simulink model "io306"  (Simulink 6.0)
settings: Solver=FixedStepDiscrete  StartTime=0.0  StopTime=4  FixedStep=0.001  RelTol=1e-3
libraries: xpcrealtimedeviceslib x6
settings Model: Creator=pkirwin  LastModifiedBy=ekbas  ExtModeArmWhenConnect=off  BufferReuse=off  ProdHWDeviceType=Specified
settings DataIOCC: SaveFormat=Structure  SignalLoggingName=sigsOut
settings OptimizationCC: BlockReduction=off  BooleanDataType=off  InlineInvariantSignals=off  OptimizeBlockIOStorage=off  BufferReuse=off  EnforceIntegerDowncast=off  FoldNonRolledExpr=off  LocalBlockOutputs=off
settings DebuggingCC: CheckExecutionContextPreStartOutputMsg=on  CheckExecutionContextRuntimeOutputMsg=on  SolverPrmCheckMsg=none
settings HardwareCC: ProdBitPerShort=32  ProdBitPerInt=16  ProdHWDeviceType=Specified  TargetHWDeviceType=32-bit Generic  ProdEqTarget=off
settings RTWCC: SystemTargetFile=xpctarget.tlc  TemplateMakefile=xpc_default_tmf  ProcessScript=xpctarget_make_rtw_hook
settings xpcTargetCC: TargetFcnLib=ansi_tfl_tmw.mat  GenFloatMathFcnCalls=ANSI_C  ModelReferenceCompliant=off
settings SFSimCC: SFSimApplyToAllLibs=on  SFSimBuildMode=Incremental

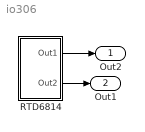
== system io306 ==
  RTD6814 : Subsystem  PropExecContextAcrossSSBoundary=on
  Out2 : Outport
  Out1 : Outport  Port=2
  wires:
  RTD6814/1(Out1) -> Out2/1
  RTD6814/2(Out2) -> Out1/1

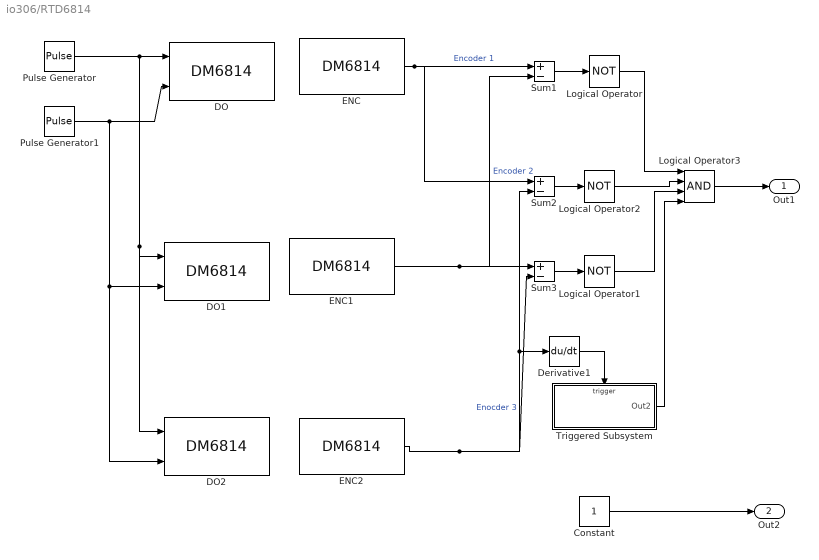
== system io306/RTD6814 ==
  Constant : Constant
  DO : xpcrealtimedeviceslib/Digital Output/DM6814   channel=[1 2]  port=A  reset=[1]  initValue=[0]  sampleTime=.001  baseHex=0x280
  DO1 : xpcrealtimedeviceslib/Digital Output/DM6814   channel=[1 2]  port=B  reset=[1]  initValue=[0]  sampleTime=.001  baseHex=0x280
  DO2 : xpcrealtimedeviceslib/Digital Output/DM6814   channel=[1 2]  port=C  reset=[1]  initValue=[0]  sampleTime=.001  baseHex=0x280
  Derivative1 : Derivative
  ENC : xpcrealtimedeviceslib/Incremental Encoder/DM6814   channel=1  initValue=0  reset=off  sampleTime=0.001  baseHex=0x280
  ENC1 : xpcrealtimedeviceslib/Incremental Encoder/DM6814   channel=2  initValue=0  reset=off  sampleTime=0.001  baseHex=0x280
  ENC2 : xpcrealtimedeviceslib/Incremental Encoder/DM6814   channel=3  initValue=0  reset=off  sampleTime=0.001  baseHex=0x280
  Logical Operator : Logic  Operator=NOT  AllPortsSameDT=off
  Logical Operator1 : Logic  Operator=NOT  AllPortsSameDT=off
  Logical Operator2 : Logic  Operator=NOT  AllPortsSameDT=off
  Logical Operator3 : Logic  Inputs=4  AllPortsSameDT=off
  Pulse Generator : DiscretePulseGenerator  Period=6000  PulseWidth=3000  PhaseDelay=500  SampleTime=0.001
  Pulse Generator1 : DiscretePulseGenerator  Period=6000  PulseWidth=3000  PhaseDelay=2500  SampleTime=0.001  VectorParams1D=off
  Sum1 : Sum  Inputs=+-  SaturateOnIntegerOverflow=on
  Sum2 : Sum  Inputs=+-  SaturateOnIntegerOverflow=on
  Sum3 : Sum  Inputs=+-  SaturateOnIntegerOverflow=on
  Triggered Subsystem : Subsystem  TreatAsAtomicUnit=on  PropExecContextAcrossSSBoundary=on
  Out1 : Outport
  Out2 : Outport  Port=2
  wires:
  Pulse Generator1/1 -> DO1/2, DO2/2, DO/2
  Pulse Generator/1 -> DO/1, DO1/1, DO2/1
  ENC/1 -> Sum1/1, Sum2/1  "Encoder 1"
  Sum1/1 -> Logical Operator/1
  ENC1/1 -> Sum3/1, Sum1/2  "Encoder 2"
  Sum3/1 -> Logical Operator1/1
  ENC2/1 -> Sum3/2, Derivative1/1, Sum2/2  "Enocder 3"
  Logical Operator/1 -> Logical Operator3/1
  Logical Operator3/1 -> Out1/1
  Sum2/1 -> Logical Operator2/1
  Logical Operator1/1 -> Logical Operator3/3
  Logical Operator2/1 -> Logical Operator3/2
  Derivative1/1 -> Triggered Subsystem/Trigger
  Constant/1 -> Out2/1
  Triggered Subsystem/1(Out2) -> Logical Operator3/4

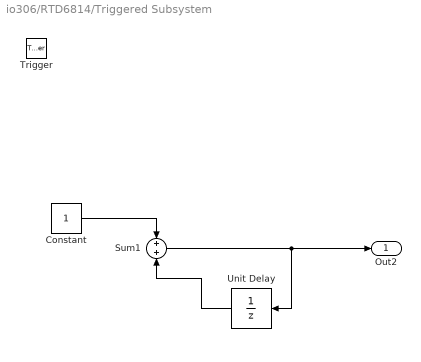
== system io306/RTD6814/Triggered Subsystem ==
  Trigger : TriggerPort
  Constant : Constant
  Sum1 : Sum  SaturateOnIntegerOverflow=on
  Unit Delay : UnitDelay  Orientation=left  X0=1  SampleTime=-1
  Out2 : Outport
  wires:
  Constant/1 -> Sum1/1
  Sum1/1 -> Out2/1, Unit Delay/1
  Unit Delay/1 -> Sum1/2
